simulink model "simModel_closed_loop_systems"  (R2025b)
settings: Solver=FixedStepAuto  StartTime=0.0  StopTime=2  FixedStep=0.001  RelTol=1e-3
InitFcn:
  | load data\FC1.mat
  | load data\FC2.mat
  | load data\FC3.mat
  | load data\FC4.mat
undefined symbols (not defined in the file or in its folder): FC1, FC2, FC3, FC4
settings Model: Creator=ismet  LastModifiedBy=ismet

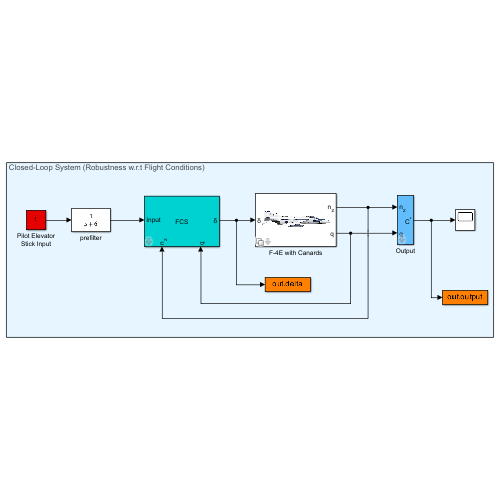
[thumbnail: Simulink's stored preview of the top-level diagram]
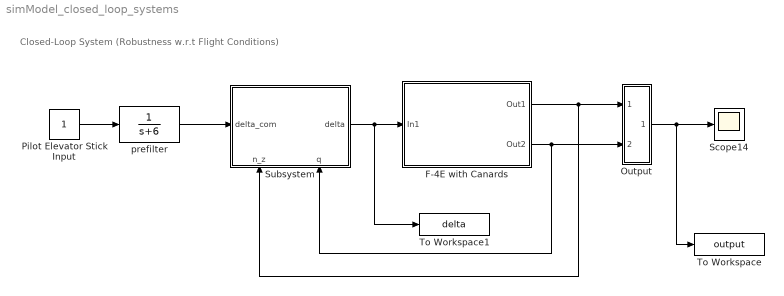
== system simModel_closed_loop_systems ==
  note: Closed-Loop System (Robustness w.r.t Flight Conditions)
  F-4E with Canards : Subsystem  Variant=on  mask{FCSelection=FC1}
      mask prompts: FCSelection "Select flight condition"
      mask TypeOptions FCSelection: FC1 | FC2 | FC3 | FC4
      mask DialogControl DescGroupVar Prompt: F4-E Aircraft with Horizontal Canards
      mask DialogControl DescTextVar Prompt: This block contains short period longitudinal mode of an F4-E aircraft with additional horizontal canards.
      mask DialogControl Control3_copy Prompt: x_dot = Ax + Bu
      mask DialogControl Control3 Prompt: State Vector: x = [n_z, q, δ_e]
      mask DialogControl Control3_copy_copy Prompt: Input: u = δ_com
      mask DialogControl ParameterGroupVar Prompt: Flight Conditions
      mask DialogControl DescTextVar_copy Prompt: There are 4 flight conditions (FCs).
      mask DialogControl DescTextVar_copy_copy Prompt: FC1: 0.5   MACH, 5000'   Altitude
      mask DialogControl DescTextVar_copy_copy_copy Prompt: FC2: 0.85 MACH, 5000'   Altitude
      mask DialogControl DescTextVar_copy_copy_copy_copy Prompt: FC3: 0.9   MACH, 35000' Altitude
      mask DialogControl DescTextVar_copy_copy_copy_copy_copy Prompt: FC4: 1.5   MACH, 35000' Altitude
      mask Display:
      | port_label('input', 1, '\delta', 'texmode', 'on');
      | port_label('output', 1, 'n_z', 'texmode', 'on');
      | port_label('output', 2, 'q', 'texmode', 'on');
      | image('.\images\F4-E-block-image.png');
  Output : Subsystem  mask{blk_c_n_z=1, blk_c_q=12.43, blk_c_c_inf=-1}
      mask prompts: blk_c_n_z "Gain for n_z"; blk_c_q "Gain for q"; blk_c_c_inf "Divider (C^inf)"
      mask DialogControl DescGroupVar Prompt: Output Measurement
      mask DialogControl DescTextVar Prompt: This is a block for obtain output to evaluate system performance.
      mask Display:
      | port_label('input', 1, 'n_z', 'texmode', 'on');
      | port_label('input', 2, 'q', 'texmode', 'on');
      | port_label('output', 1, 'C^*', 'texmode', 'on');
  Pilot Elevator Stick Input : Constant
  Scope14 : Scope
      settings: ActiveDisplayYMinimum=-1.7819501620372069  ActiveDisplayYMaximum=16.037551458334868  DataLoggingVariableName=ScopeData14
  Subsystem : Subsystem  mask{blk_k_n_z=-0.115, blk_k_q=-0.8}
      mask prompts: blk_k_n_z "Gain for n_z"; blk_k_q "Gain for    q"
      settings: PortSchema="{\"entries\":[{\"content\":{\"sides\":[{\"content\":{\"connectorIds\":[\"In1\"]},\"type\":\"ConnectorPlacement.EquallySpacedRectSide\",\"uuid\":\"39ad9b64-1b92-4a0c-81c1-7d2facf88cb6\"},{\"content\":{\"connectorIds\":[\"Out1\"],\"side\":\"RIGHT\"},\"type\":\"ConnectorPlacement.EquallySpacedRectSide\",\"uuid\":\"5abddeba-1daf-4d66-a884-f1939584c310\"},{\"content\":{\"side\":\"TOP\"},\"type\":\"ConnectorPlacement.EquallySpacedRectSide\",\"uuid\":\"152bc167-3377-450d-a2a5-1c8b1bc05f21\"},{\"content\":{\"connectorIds\":[\"In2\",\"In3\"],\"side\":\"BOTTOM\"},\"type\":\"ConnectorPlacement.EquallySpacedRectSide\",\"uuid\":\"90770360-401c-43fc-8324-5236ed2b29ff\"}]},\"type\":\"ConnectorPlacement.EquallySpacedConnector\",\"uuid\":\"237a1dba-7a82-4433-a5f1-292fcb4a53bd\"}],\"packageUris\":[\"http://schema.mathworks.com/mf0/Connector/R2020b\"],\"version\":\"1.0\"}"
      mask DialogControl DescGroupVar Prompt: Flight Controller for F4-E
      mask DialogControl DescTextVar Prompt: This is a state-feedback controller implementation.
      mask DialogControl ParameterGroupVar Prompt: Controller Parameters
      mask Display:
      | port_label('input', 1, 'Input');
      | port_label('input', 2, 'n_z', 'texmode', 'on');
      | port_label('input', 3, 'q', 'texmode', 'on');
      | port_label('output', 1, '\delta', 'texmode', 'on');
      | 
      | disp('FCS');
  To Workspace : ToWorkspace  VariableName=output  SaveFormat=Timeseries  SampleTime=-1
  To Workspace1 : ToWorkspace  VariableName=delta  SaveFormat=Timeseries  SampleTime=-1
  prefilter : TransferFcn  Denominator=[1 6]
  wires:
  F-4E with Canards/1(Out1) -> Subsystem/2(n_z), Output/1(n_z)
  F-4E with Canards/2(Out2) -> Subsystem/3(q), Output/2(q)
  Output/1(C*) -> To Workspace/1, Scope14/1
  Pilot Elevator Stick Input/1 -> prefilter/1
  Subsystem/1(delta) -> To Workspace1/1, F-4E with Canards/1(In1)
  prefilter/1 -> Subsystem/1(delta_com)

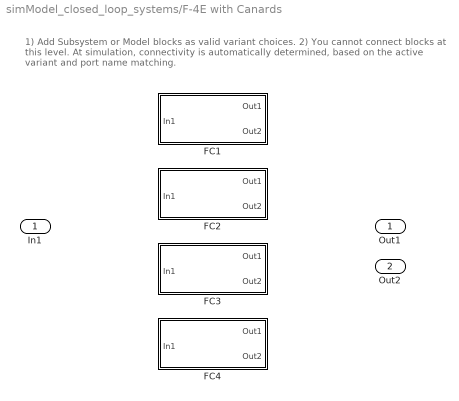
== system simModel_closed_loop_systems/F-4E with Canards ==
  note: 1) Add Subsystem or Model blocks as valid variant choices.
      | 2) You cannot connect blocks at this level. At simulation, connectivity is automatically
      | determined, based on the active variant and port name matching.
  In1 : Inport
  FC1 : Subsystem  VariantControl="FCSelection == \"FC1\""
  FC2 : Subsystem  VariantControl="FCSelection == \"FC2\""
  FC3 : Subsystem  VariantControl="FCSelection == \"FC3\""
  FC4 : Subsystem  VariantControl="FCSelection == \"FC4\""
  Out1 : Outport
  Out2 : Outport  Port=2

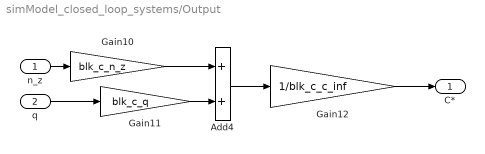
== system simModel_closed_loop_systems/Output ==
  n_z : Inport
  q : Inport  Port=2
  Add4 : Sum
  Gain10 : Gain  Gain=blk_c_n_z
  Gain11 : Gain  Gain=blk_c_q
  Gain12 : Gain  Gain=1/blk_c_c_inf
  C* : Outport
  wires:
  n_z/1 -> Gain10/1
  Gain10/1 -> Add4/1
  Add4/1 -> Gain12/1
  Gain11/1 -> Add4/2
  Gain12/1 -> C*/1
  q/1 -> Gain11/1

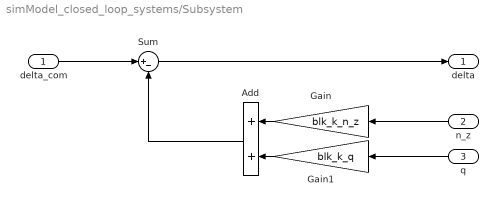
== system simModel_closed_loop_systems/Subsystem ==
  delta_com : Inport
  n_z : Inport  Port=2
  q : Inport  Port=3
  Add : Sum
  Gain : Gain  Gain=blk_k_n_z
  Gain1 : Gain  Gain=blk_k_q
  Sum : Sum  Inputs=|+-
  delta : Outport
  wires:
  q/1 -> Gain1/1
  n_z/1 -> Gain/1
  Sum/1 -> delta/1
  delta_com/1 -> Sum/1
  Gain1/1 -> Add/2
  Gain/1 -> Add/1
  Add/1 -> Sum/2

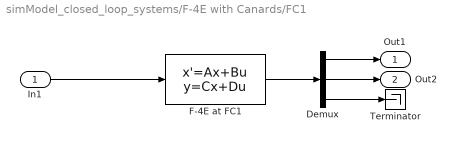
== system simModel_closed_loop_systems/F-4E with Canards/FC1 ==
  In1 : Inport
  Demux : Demux  Outputs=3
  F-4E at FC1 : StateSpace  A=FC1.A  B=FC1.B  C=FC1.C  D=FC1.D  InitialCondition=0  ContinuousStateAttributes=['n_z', 'q', 'delta_e']
  Terminator : Terminator
  Out1 : Outport
  Out2 : Outport  Port=2
  wires:
  In1/1 -> F-4E at FC1/1
  F-4E at FC1/1 -> Demux/1
  Demux/1 -> Out1/1
  Demux/2 -> Out2/1
  Demux/3 -> Terminator/1

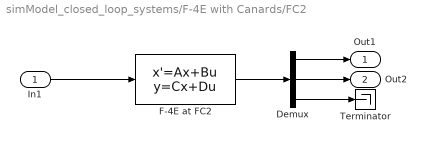
== system simModel_closed_loop_systems/F-4E with Canards/FC2 ==
  In1 : Inport
  Demux : Demux  Outputs=3
  F-4E at FC2 : StateSpace  A=FC2.A  B=FC2.B  C=FC2.C  D=FC2.D  InitialCondition=0  ContinuousStateAttributes=['n_z', 'q', 'delta_e']
  Terminator : Terminator
  Out1 : Outport
  Out2 : Outport  Port=2
  wires:
  In1/1 -> F-4E at FC2/1
  Demux/1 -> Out1/1
  Demux/3 -> Terminator/1
  F-4E at FC2/1 -> Demux/1
  Demux/2 -> Out2/1

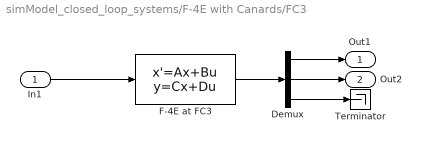
== system simModel_closed_loop_systems/F-4E with Canards/FC3 ==
  In1 : Inport
  Demux : Demux  Outputs=3
  F-4E at FC3 : StateSpace  A=FC3.A  B=FC3.B  C=FC3.C  D=FC3.D  InitialCondition=0  ContinuousStateAttributes=['n_z', 'q', 'delta_e']
  Terminator : Terminator
  Out1 : Outport
  Out2 : Outport  Port=2
  wires:
  In1/1 -> F-4E at FC3/1
  Demux/1 -> Out1/1
  Demux/3 -> Terminator/1
  F-4E at FC3/1 -> Demux/1
  Demux/2 -> Out2/1

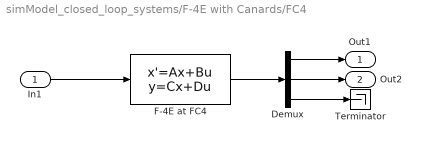
== system simModel_closed_loop_systems/F-4E with Canards/FC4 ==
  In1 : Inport
  Demux : Demux  Outputs=3
  F-4E at FC4 : StateSpace  A=FC4.A  B=FC4.B  C=FC4.C  D=FC4.D  InitialCondition=0  ContinuousStateAttributes=['n_z', 'q', 'delta_e']
  Terminator : Terminator
  Out1 : Outport
  Out2 : Outport  Port=2
  wires:
  In1/1 -> F-4E at FC4/1
  Demux/1 -> Out1/1
  Demux/3 -> Terminator/1
  F-4E at FC4/1 -> Demux/1
  Demux/2 -> Out2/1
